simulink model "SimulinkCircuits"  (R2019a)
settings: Solver=ode1  StartTime=0.0  StopTime=200  FixedStep=0.001  MaxStep=0.001  RelTol=1e-3
values from neighbouring files (symbols this model uses):
  delaypos = delayy    (= 0)    [Project.m]
  delaystation1 = 1.5    [Project.m]
  delaystation2 = 50    [Project.m]
  delaystation3 = 125    [Project.m]
  delaystation4 = 300    [Project.m]
  L = acker(sys.A',sys.C',[-4 -8 -12])'    [Project.m]
  sys = ss(A,B,C,0)    [Project.m]
  xdisp = 0    [Project.m]
  ydisp = 0    [Project.m]
libraries: cstblocks x10, simulink x9
settings Model: Creator=cooper  LastModifiedBy=cooper

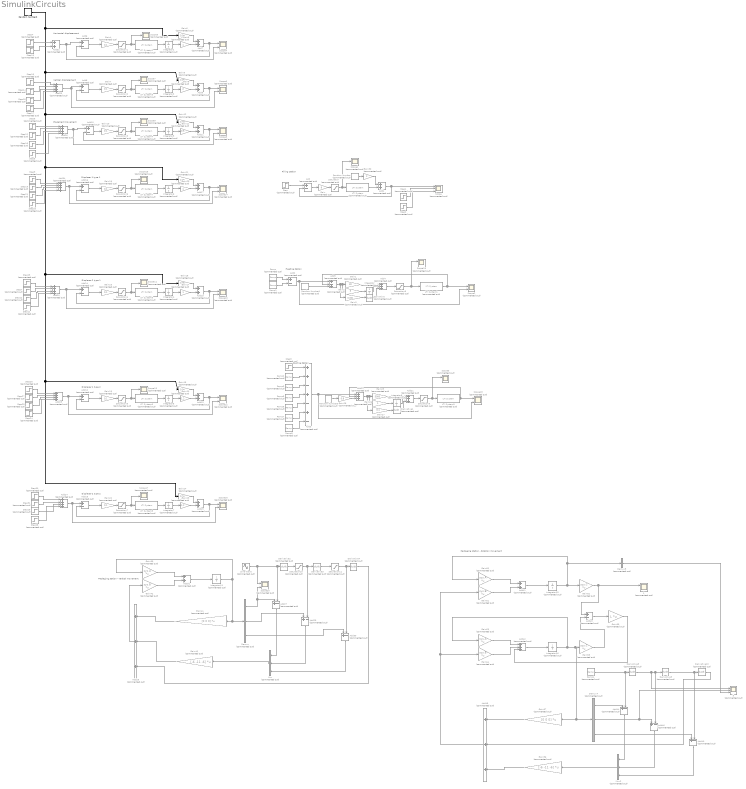
== system SimulinkCircuits ==
  note: Packaging station - Rotation movement
  note: Cooling station
  note: Heating station
  note: Filling station
  note: Horizontal displacement
  note: Vertical displacement
  note: Placement movement
  note: Displacer 2 type 1
  note: Displacer 1 type 2
  note: Displacer 1 type 1
  note: Displacer 2 type 2
  note: Packaging station - Vertical movement
  " 4" : Scope  Commented=on  NumInputPorts=2
  " 5" : Scope  Commented=on  NumInputPorts=3
  Add{,2,6,8,10,12,14,16,18,27,29..30,40,43..44,46} (16 alike) : Sum  Commented=on  Inputs=+-
  Add{1,7,9,11,13,15,17,19,31..32,41} (11 alike) : Sum  Commented=on
  Add{20,23..24,26,33..34} (6 alike) : Sum  Commented=on  Inputs=++++
  Add{4,21,28,42,45} (5 alike) : Sum  Commented=on  Inputs=+++
  Add22 : Sum  Commented=on  Inputs=+-+
  Add3 : Sum  Commented=on  Inputs=++-+-+-
  Add5 : Sum  Commented=on  Inputs=+-+
  Demux : Demux  Commented=on  Outputs=3
  Demux4 : Demux  Commented=on  Outputs=3
  Demux5 : Demux  Commented=on  Outputs=3
  Derivative{,1..4,8..10} (8 alike) : Derivative  Commented=on
  Gain : Gain  Commented=on  Gain=8
  Gain1 : Gain  Commented=on  Gain=30
  Gain{4,7,10,13,16,19,22,27} (8 alike) : Gain  Commented=on  Gain=0.1
  Gain11 : Gain  Commented=on  Gain=0.5
  Gain12 : Gain  Commented=on  Gain=0.03
  Gain14 : Gain  Commented=on  Gain=1.2
  Gain15 : Gain  Commented=on  Gain=0.04
  Gain{5,17,20,26} (4 alike) : Gain  Commented=on
  Gain18 : Gain  Commented=on  Gain=0.05
  Gain2 : Gain  Commented=on  Gain=3
  Gain21 : Gain  Commented=on  Gain=0.05
  Gain23 : Gain  Commented=on  Gain=1.2
  Gain24 : Gain  Commented=on  Gain=0.04
  Gain25 : Gain  Commented=on  Gain=5000
  Gain28 : Gain  Commented=on  Gain=0.8
  Gain3 : Gain  Commented=on  Gain=0.001
  Gain30 : Gain  Commented=on  Gain=2
  Gain39 : Gain  Commented=on  Gain=sys.A  Multiplication=Matrix(K*u)
  Gain40 : Gain  Commented=on  Gain=[-6 -11 -6]  Multiplication=Matrix(K*u)
  Gain41 : Gain  Commented=on  Gain=[0 0 0]  Multiplication=Matrix(K*u)
  Gain42 : Gain  Commented=on  Gain=sys.B  Multiplication=Matrix(K*u)
  Gain56 : Gain  Commented=on  Gain=[-6 -11 -6]  Multiplication=Matrix(K*u)
  Gain57 : Gain  Commented=on  Gain=[0 0 0]  Multiplication=Matrix(K*u)
  Gain58 : Gain  Commented=on  Gain=sys.C  Multiplication=Matrix(K*u)
  Gain59 : Gain  Commented=on  Gain=L  Multiplication=Matrix(K*u)
  Gain6 : Gain  Commented=on  Gain=0.04
  Gain60 : Gain  Commented=on  Gain=sys.A  Multiplication=Matrix(K*u)
  Gain61 : Gain  Commented=on  Gain=sys.B  Multiplication=Matrix(K*u)
  Gain62 : Gain  Commented=on  Gain=sys.C  Multiplication=Matrix(K*u)
  Gain63 : Gain  Commented=on  Gain=sys.A  Multiplication=Matrix(K*u)
  Gain64 : Gain  Commented=on  Gain=sys.B  Multiplication=Matrix(K*u)
  Gain8 : Gain  Commented=on  Gain=2
  Gain9 : Gain  Commented=on  Gain=0.05
  Integrator{,1..8} (9 alike) : Integrator  Commented=on
  Integrator11 : Integrator  Commented=on  InitialCondition=-10
  Integrator15 : Integrator  Commented=on  InitialCondition=[1 0.2 0.3]
  Integrator16 : Integrator  Commented=on  InitialCondition=[-1 0.2 0.5]
  LTI System : cstblocks/LTI System  Commented=on  sys=tf(1,[1 0])  IC=[]
  LTI System1 : cstblocks/LTI System  Commented=on  sys=tf(325,[12 1])  IC=[]
  LTI System{2..8} (7 alike) : cstblocks/LTI System  Commented=on  sys=G  IC=[]
  LTI System9 : cstblocks/LTI System  Commented=on  sys=tf(240,[8 1])  IC=[]
  Mux : Mux  Commented=on  Inputs=3
  Mux2 : Mux  Commented=on  Inputs=3
  Ramp : simulink/Sources/Ramp  Commented=on  slope=10  start=0  InitialOutput=0
  Ramp1 : simulink/Sources/Ramp  Commented=on  slope=10  start=20  InitialOutput=0
  Ramp2 : simulink/Sources/Ramp  Commented=on  slope=-3  start=0  InitialOutput=0
  Ramp3 : simulink/Sources/Ramp  Commented=on  slope=-3  start=20  InitialOutput=0
  Ramp4 : simulink/Sources/Ramp  Commented=on  slope=50  start=0  InitialOutput=0
  Ramp5 : simulink/Sources/Ramp  Commented=on  slope=-4  start=40  InitialOutput=0
  Ramp6 : simulink/Sources/Ramp  Commented=on  slope=-4  start=60  InitialOutput=0
  Ramp7 : simulink/Sources/Ramp  Commented=on  slope=-5  start=80  InitialOutput=0
  Ramp8 : simulink/Sources/Ramp  Commented=on  slope=-5  start=90  InitialOutput=0
  Random Number : RandomNumber  Commented=on  SampleTime=0.001
  Random Number1 : RandomNumber  Commented=on  SampleTime=0.001
  Random Number2 : RandomNumber  SampleTime=0.001
  Random Number3 : RandomNumber  Commented=on  SampleTime=0.001
  Saturation : Saturate  Commented=on  UpperLimit=250
  Saturation{1..7} (7 alike) : Saturate  Commented=on  UpperLimit=0.9  LowerLimit=-0.9
  Saturation10 : Saturate  Commented=on  UpperLimit=20  LowerLimit=-20
  Saturation11 : Saturate  Commented=on  UpperLimit=20  LowerLimit=-20
  Saturation8 : Saturate  Commented=on  UpperLimit=1  LowerLimit=0
  Saturation9 : Saturate  Commented=on  UpperLimit=0  LowerLimit=-1
  Scope : Scope  Commented=on  NumInputPorts=3
  Scope{1,5,7,9,11,13,15,17} (8 alike) : Scope  Commented=on
  Scope{2..4,6,8,10,12,14,16,18..20} (12 alike) : Scope  Commented=on  NumInputPorts=2
  Sine Wave : Sin  Commented=on  Amplitude=10  Frequency=2*pi/60  SampleTime=0
  Step : Step  Commented=on  Time=0  After=250  SampleTime=0
  Step1 : Step  Commented=on  Time=0  After=245  SampleTime=0
  Step11 : Step  Commented=on  Time=30+2+30+delaystation2+30+2  After=-30  SampleTime=0
  Step12 : Step  Commented=on  Time=delaypos+50  After=15  SampleTime=0
  Step13 : Step  Commented=on  Time=delaypos+100  After=-xdisp  SampleTime=0
  Step14 : Step  Commented=on  Time=delaypos+100  After=-ydisp  SampleTime=0
  Step15 : Step  Commented=on  Time=0  After=ydisp  SampleTime=0
  Step16 : Step  Commented=on  Time=2*delaypos+100  After=25  SampleTime=0
  Step17 : Step  Commented=on  Time=2*delaypos+100+60+10  SampleTime=0
  Step18 : Step  Commented=on  Time=2*delaypos+100+60  After=-1  SampleTime=0
  Step{7,19,27,31} (4 alike) : Step  Commented=on  Time=30+2  After=-30  SampleTime=0
  Step2 : Step  Commented=on  Time=0  After=260  SampleTime=0
  Step20 : Step  Commented=on  Time=30+2+30+delaystation1+30+2  After=-30  SampleTime=0
  Step21 : Step  Commented=on  Time=30+2+30+delaystation1  After=30  SampleTime=0
  Step22 : Step  Commented=on  Time=30+2+30+delaystation2  After=30  SampleTime=0
  Step{9,23,26,30} (4 alike) : Step  Commented=on  Time=0  After=30  SampleTime=0
  Step24 : Step  Commented=on  Time=30+2+30+delaystation3+30+2  After=-30  SampleTime=0
  Step25 : Step  Commented=on  Time=30+2+30+delaystation3  After=30  SampleTime=0
  Step28 : Step  Commented=on  Time=30+2+30+delaystation4+30+2  After=-30  SampleTime=0
  Step29 : Step  Commented=on  Time=30+2+30+delaystation4  After=30  SampleTime=0
  Step3 : Step  Commented=on  Time=0  After=0  SampleTime=0
  Step4 : Step  Commented=on  Time=0  After=xdisp  SampleTime=0
  Step5 : Step  Commented=on  Time=2*delaypos+100+60+20  After=-25  SampleTime=0
  Step6 : Step  Commented=on  Time=delaypos  After=-15  SampleTime=0
  wires:
  Add/1 -> Gain/1
  Step/1 -> Add/1
  Step1/1 -> Scope/2
  Step2/1 -> Scope/3
  LTI System/1 -> Add1/2
  Gain/1 -> Saturation/1
  Saturation/1 -> Scope1/1, LTI System/1
  Add1/1 -> Add/2, Scope/1
  Gain1/1 -> Add4/1
  Ramp/1 -> Add2/1
  Ramp1/1 -> Add2/2
  Gain2/1 -> Integrator/1
  Gain3/1 -> Derivative/1
  Add5/1 -> Gain3/1, Gain2/1, Gain1/1
  Integrator/1 -> Add4/2
  Derivative/1 -> Add4/3
  Add2/1 -> Scope2/2, Add5/1
  LTI System1/1 -> Add5/2, Scope2/1
  Step3/1 -> Add3/1
  Ramp2/1 -> Add3/2
  Ramp3/1 -> Add3/3
  Ramp5/1 -> Add3/4
  Ramp6/1 -> Add3/5
  Ramp7/1 -> Add3/6
  Ramp8/1 -> Add3/7
  Add6/1 -> Gain4/1
  LTI System2/1 -> Integrator1/1
  Integrator1/1 -> Gain5/1
  Gain5/1 -> Add7/2
  Gain6/1 -> Add7/1
  Add7/1 -> Scope4/1, Add6/2
  Gain4/1 -> Saturation1/1
  Saturation1/1 -> Scope5/1, LTI System2/1
  Saturation2/1 -> LTI System3/1, Scope7/1
  Gain7/1 -> Saturation2/1
  Add9/1 -> Add8/2, Scope6/1
  Gain9/1 -> Add9/1
  Gain8/1 -> Add9/2
  Integrator2/1 -> Gain8/1
  LTI System3/1 -> Integrator2/1
  Add8/1 -> Gain7/1
  Add33/1 -> Add8/1, Scope6/2
  Random Number2/1 -> Gain6/1, Gain12/1, Gain21/1, Gain18/1, Gain15/1, Gain24/1, Gain9/1
  Add10/1 -> Gain10/1
  LTI System4/1 -> Integrator3/1
  Integrator3/1 -> Gain11/1
  Gain11/1 -> Add11/2
  Gain12/1 -> Add11/1
  Add11/1 -> Scope8/1, Add10/2
  Gain10/1 -> Saturation3/1
  Saturation3/1 -> Scope9/1, LTI System4/1
  Saturation5/1 -> LTI System6/1, Scope13/1
  Gain13/1 -> Saturation5/1
  Add13/1 -> Add12/2, Scope12/1
  Gain15/1 -> Add13/1
  Gain14/1 -> Add13/2
  Integrator5/1 -> Gain14/1
  LTI System6/1 -> Integrator5/1
  Add12/1 -> Gain13/1
  Add14/1 -> Gain16/1
  LTI System5/1 -> Integrator4/1
  Integrator4/1 -> Gain17/1
  Gain17/1 -> Add15/2
  Gain18/1 -> Add15/1
  Add15/1 -> Scope10/1, Add14/2
  Gain16/1 -> Saturation4/1
  Saturation4/1 -> Scope11/1, LTI System5/1
  Saturation6/1 -> LTI System7/1, Scope15/1
  Gain19/1 -> Saturation6/1
  Add17/1 -> Add16/2, Scope14/1
  Gain21/1 -> Add17/1
  Gain20/1 -> Add17/2
  Integrator6/1 -> Gain20/1
  LTI System7/1 -> Integrator6/1
  Add16/1 -> Gain19/1
  Add18/1 -> Gain22/1
  LTI System8/1 -> Integrator7/1
  Integrator7/1 -> Gain23/1
  Gain23/1 -> Add19/2
  Gain24/1 -> Add19/1
  Add19/1 -> Scope16/1, Add18/2
  Gain22/1 -> Saturation7/1
  Saturation7/1 -> Scope17/1, LTI System8/1
  LTI System9/1 -> Add22/2, Scope18/1
  Derivative1/1 -> Add21/3
  Integrator8/1 -> Add21/2
  Add22/1 -> Gain25/1, Gain26/1, Gain27/1
  Gain27/1 -> Derivative1/1
  Gain26/1 -> Integrator8/1
  Gain25/1 -> Add21/1
  Random Number3/1 -> Gain28/1
  Add21/1 -> Saturation9/1
  Saturation9/1 -> Scope3/1, LTI System9/1
  Add30/1 -> Mux/3
  Gain39/1 -> Add31/1  "Ax"
  Gain40/1 -> Add28/2
  Derivative2/1 -> Saturation10/1
  Derivative3/1 -> Saturation11/1
  Mux/1 -> Gain40/1
  Sine Wave/1 -> Add27/2, Derivative2/1, Scope20/1
  Add28/1 -> Gain42/1  "u"
  Add29/1 -> Mux/2
  Derivative4/1 -> Add28/3
  Saturation10/1 -> Derivative3/1, Add29/2
  Demux/1 -> Scope20/2, Add27/1
  Gain41/1 -> Add28/1
  Add27/1 -> Mux/1
  Add31/1 -> Integrator11/1  "dx"
  Saturation11/1 -> Add30/2, Derivative4/1
  Gain42/1 -> Add31/2  "Bu"
  Integrator11/1 -> Gain41/1, Demux/1, Gain39/1  "x"
  Demux/3 -> Add30/1
  Demux/2 -> Add29/1
  Add41/1 -> Integrator15/1  "dx"
  Ramp4/1 -> Add44/2, Derivative8/1
  Mux2/1 -> Gain56/1
  Gain58/1 -> Add43/2  "s"
  Add46/1 -> Mux2/2
  Gain59/1 -> Add42/3
  Integrator16/1 -> Demux4/1, Gain57/1, Gain58/1, Gain63/1  "o"
  Derivative10/1 -> Add45/2
  Gain63/1 -> Add42/1  "Ax"
  Add44/1 -> Mux2/1
  Add42/1 -> Integrator16/1  "do"
  Gain56/1 -> Add45/3
  Derivative9/1 -> Add40/2, Derivative10/1
  Add43/1 -> Gain59/1  "y-s"
  Gain61/1 -> Add41/2  "Bu"
  Gain62/1 -> " 4"/1, Add43/1  "y"
  Derivative8/1 -> " 5"/1, Derivative9/1, Add46/2
  Gain60/1 -> Add41/1  "Ax"
  Gain64/1 -> Add42/2  "Bu"
  Gain57/1 -> Add45/1
  Demux4/1 -> Add44/1
  Demux4/2 -> " 5"/2, Add46/1
  Add45/1 -> Gain64/1, Gain61/1  "u"
  Add40/1 -> Mux2/3
  Integrator15/1 -> Gain62/1, Gain60/1, Demux5/1  "x"
  Demux4/3 -> Add40/1
  Demux5/2 -> " 5"/3
  Step6/1 -> Add26/1
  Step12/1 -> Add26/2
  Step4/1 -> Add32/1
  Step13/1 -> Add32/2
  Add32/1 -> Scope4/2, Add6/1
  Step14/1 -> Add33/2
  Step15/1 -> Add33/1
  Add26/1 -> Scope8/2, Add10/1
  Step16/1 -> Add26/3
  Step5/1 -> Add26/4
  Step18/1 -> Add33/3
  Step17/1 -> Add33/4
  Add3/1 -> Scope18/2, Add22/1
  Step9/1 -> Add34/1
  Step19/1 -> Add34/2
  Add34/1 -> Scope14/2, Add16/1
  Step21/1 -> Add34/3
  Step20/1 -> Add34/4
  Step11/1 -> Add20/4
  Step22/1 -> Add20/3
  Step7/1 -> Add20/2
  Step23/1 -> Add20/1
  Step26/1 -> Add23/1
  Step27/1 -> Add23/2
  Step25/1 -> Add23/3
  Step24/1 -> Add23/4
  Step28/1 -> Add24/4
  Step29/1 -> Add24/3
  Step31/1 -> Add24/2
  Step30/1 -> Add24/1
  Add24/1 -> Scope16/2, Add18/1
  Add23/1 -> Scope12/2, Add12/1
  Add20/1 -> Scope10/2, Add14/1
  Random Number/1 -> Gain30/1
  Gain30/1 -> Add1/1
  Add4/1 -> Saturation8/1
  Saturation8/1 -> Scope19/1, LTI System1/1
  Random Number1/1 -> Add5/3
  Gain28/1 -> Add22/3
